simulink model "instalatie"  (R2022b)
settings: Solver=VariableStepAuto  StartTime=0.0  StopTime=10.0  RelTol=1e-3
settings Model: Creator=fabian  LastModifiedBy=fabian

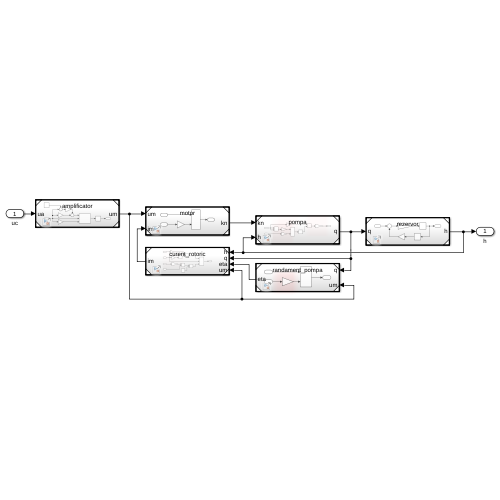
[thumbnail: Simulink's stored preview of the top-level diagram]
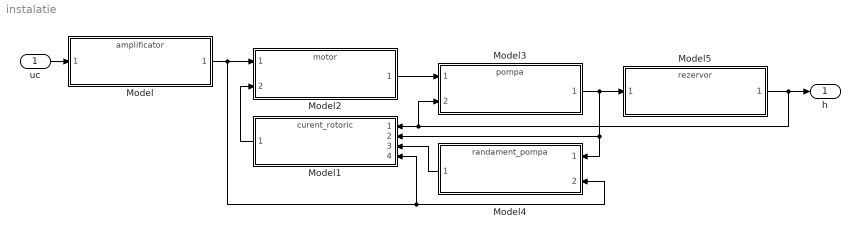
== system instalatie ==
  uc : Inport
  Model : ModelReference  ModelNameDialog=amplificator.slx  SimulationMode=Normal  ModelReferenceVersion=1.1
  Model1 : ModelReference  ModelNameDialog=curent_rotoric.slx  SimulationMode=Normal  ModelReferenceVersion=1.2
  Model2 : ModelReference  ModelNameDialog=motor.slx  SimulationMode=Normal  ModelReferenceVersion=1.1
  Model3 : ModelReference  ModelNameDialog=pompa.slx  SimulationMode=Normal  ModelReferenceVersion=1.1
  Model4 : ModelReference  ModelNameDialog=randament_pompa.slx  SimulationMode=Normal  ModelReferenceVersion=1.1
  Model5 : ModelReference  ModelNameDialog=rezervor.slx  SimulationMode=Normal  ModelReferenceVersion=1.1
  h : Outport
  wires:
  uc/1 -> Model/1
  Model/1 -> Model2/1, Model1/4, Model4/2
  Model2/1 -> Model3/1
  Model3/1 -> Model5/1, Model4/1, Model1/2
  Model5/1 -> h/1, Model3/2, Model1/1
  Model1/1 -> Model2/2
  Model4/1 -> Model1/3
